simulink model "simulator"  (R2023b)
settings: Solver=VariableStepAuto  StartTime=0.0  StopTime=20  RelTol=1e-3
libraries: fuzblock x1
settings Model: Creator=lima  LastModifiedBy=diogo
settings SolverCC: AlgebraicLoopSolver=TrustRegion
settings DebuggingCC: UnconnectedInputMsg=warning  UnconnectedOutputMsg=warning  UnconnectedLineMsg=warning
settings ModelReferenceCC: EnableRefExpFcnMdlSchedulingChecks=on
settings RTWCC: DLArmComputeVersion=19.05

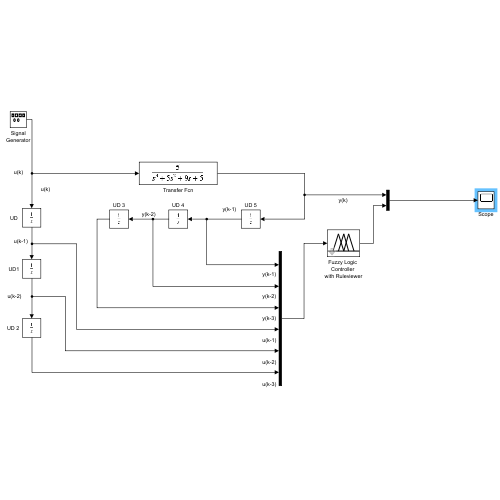
[thumbnail: Simulink's stored preview of the top-level diagram]
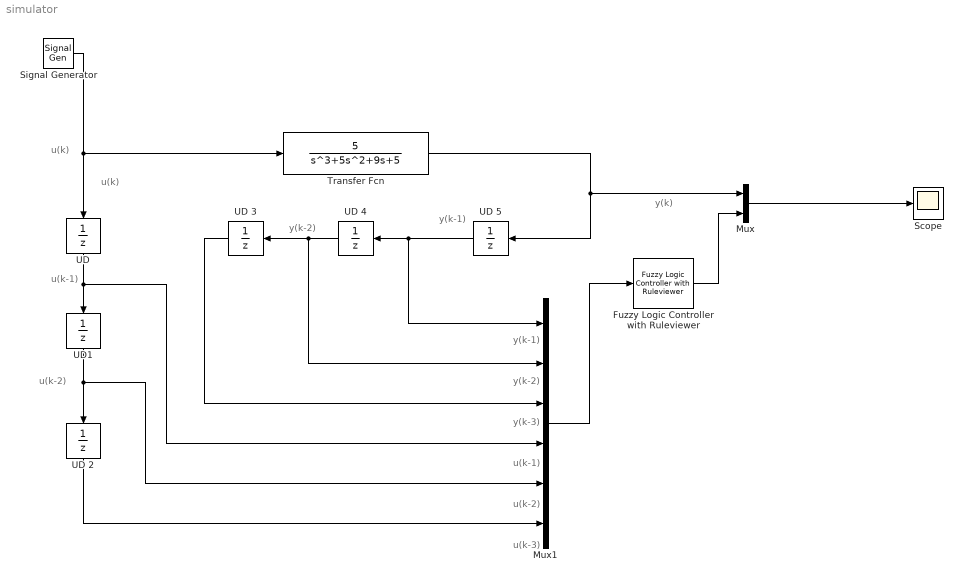
== system simulator ==
  note: u(k)
  note: u(k-3)
  note: u(k-2)
  note: u(k-1)
  note: y(k-3)
  note: y(k-2)
  note: y(k-1)
  note: y(k)
  note: u(k)
  note: u(k-1)
  note: u(k-2)
  note: y(k-1)
  note: y(k-2)
  Fuzzy Logic Controller with Ruleviewer : fuzblock/Fuzzy Logic  Controller  with Ruleviewer  fismatrix=subtractive_hybrid  Ts=0.1
  Mux : Mux  Inputs=2
  Mux1 : Mux  Inputs=6
  Scope : Scope
  Signal Generator : SignalGenerator  WaveForm=sawtooth  Units=rad/sec
  Transfer Fcn : TransferFcn  Numerator=[5]  Denominator=[1 5 9 5]
  "UD " : UnitDelay  SampleTime=0.1  HasFrameUpgradeWarning=on
  UD {2..5} (4 alike) : UnitDelay  SampleTime=-1  HasFrameUpgradeWarning=on
  UD1 : UnitDelay  SampleTime=-1  HasFrameUpgradeWarning=on
  wires:
  "UD "/1 -> Mux1/4, UD1/1
  UD1/1 -> Mux1/5, UD 2/1
  Signal Generator/1 -> "UD "/1, Transfer Fcn/1
  Transfer Fcn/1 -> UD 5/1, Mux/1
  UD 5/1 -> Mux1/1, UD 4/1
  UD 4/1 -> Mux1/2, UD 3/1
  Mux1/1 -> Fuzzy Logic Controller with Ruleviewer/1
  Fuzzy Logic Controller with Ruleviewer/1 -> Mux/2
  Mux/1 -> Scope/1
  UD 3/1 -> Mux1/3
  UD 2/1 -> Mux1/6
